simulink model "Battery_v2"  (R2024b)
settings: Solver=VariableStepAuto  StartTime=0.0  StopTime=inf  RelTol=1e-3
settings Model: Creator=miche  LastModifiedBy=miche

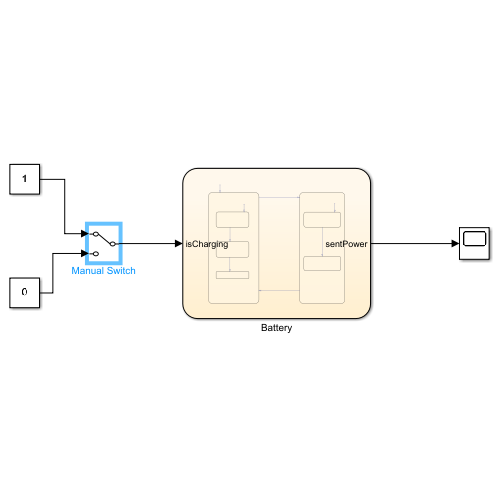
[thumbnail: Simulink's stored preview of the top-level diagram]
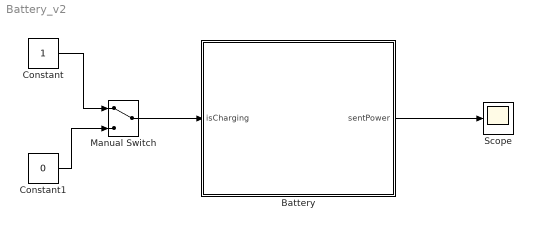
== system Battery_v2 ==
  Battery : Stateflow chart  TreatAsAtomicUnit=on
  Constant : Constant  SampleTime=0.5
  Constant1 : Constant  Value=0  SampleTime=0.5
  Manual Switch : ManualSwitch
  Scope : Scope
  wires:
  Constant/1 -> Manual Switch/1
  Constant1/1 -> Manual Switch/2
  Manual Switch/1 -> Battery/1(isCharging)
  Battery/1(sentPower) -> Scope/1

== stateflow chart Battery_v2/Battery ==
  state Charge
    entry:
    sentPower = 0;
    state FastCharge
      during:
      charge = charge +4;
    state SlowChart
      during:
      charge = charge +1
    state Full
    (default) -> FastCharge
    FastCharge -> SlowChart : [charge > 80]
    SlowChart -> Full : [charge == 100]
  state Discharge
    entry:
    sentPower = 3.5;
    state Powered
      during:
      charge = charge - 3
    state Empty
      entry:
      sentPower = 0;
    (default) -> Powered
    Powered -> Empty : [charge<=3]
  (default) -> Charge
  Charge -> Discharge : [~isCharging]
  Discharge -> Charge : [isCharging]
  data: isCharging input; sentPower output; charge local =50
